simulink model "TrainModel"  (R2021a)
settings: Solver=FixedStepAuto  StartTime=0.0  StopTime=50  FixedStep=0.01  RelTol=1e-3
StopFcn:
  | if (exist('SimulinkOutput', 'file')==2)
  | SimulinkOutput(out)
  | end
settings Model: Creator=vaibhavdeshmukh  LastModifiedBy=vdmac
settings SolverCC: AlgebraicLoopSolver=TrustRegion
settings DebuggingCC: SFMachineParentedDataDiag=warning

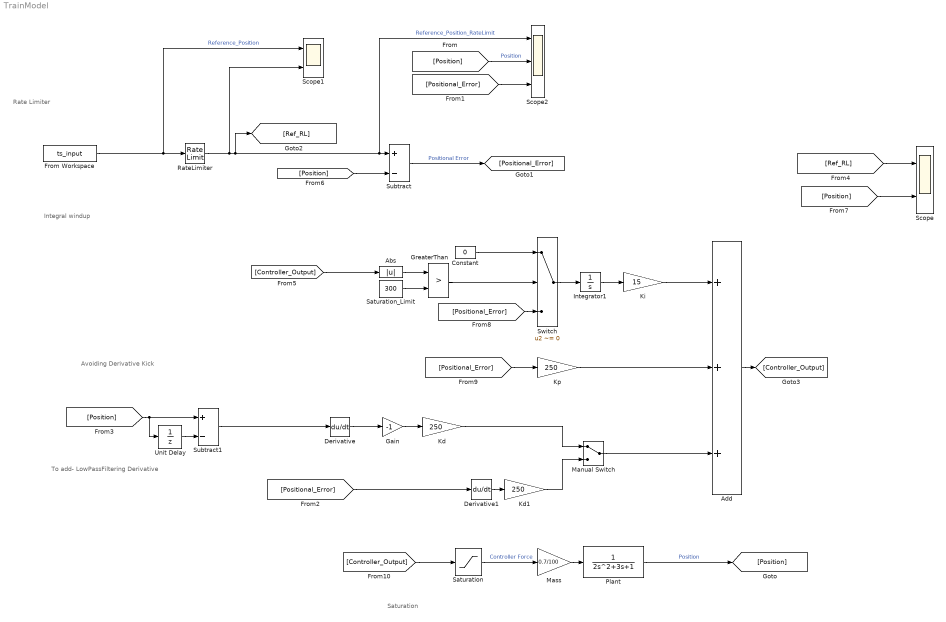
== system TrainModel ==
  note: Rate Limiter
  note: Saturation
  note: Avoiding Derivative Kick
  note: Integral windup
  note: To add- LowPassFiltering Derivative
  Abs : Abs
  Add : Sum  Inputs=+++
  Constant : Constant  Value=0
  Derivative : Derivative
  Derivative1 : Derivative
  From Workspace : FromWorkspace  VariableName=ts_input
  Gain : Gain  Gain=-1
  GreaterThan : RelationalOperator  Operator=>  OutDataTypeStr=boolean  RndMeth=Simplest
  Integrator1 : Integrator
  Kd : Gain  Gain=250
  Kd1 : Gain  Gain=250
  Ki : Gain  Gain=15
  Kp : Gain  Gain=250
  Manual Switch : ManualSwitch
  Mass : Gain  Gain=0.7/100
  Plant : TransferFcn  Denominator="[2 3  1]"
  RateLimiter : RateLimiter  RisingSlewLimit=20  FallingSlewLimit=-20  SampleTimeMode=inherited
  Saturation : Saturate  UpperLimit=10000  LowerLimit=-10000
  Saturation_Limit : Constant  Value=300
  Scope : Scope  NumInputPorts=2
  Scope1 : Scope  NumInputPorts=2
  Scope2 : Scope  NumInputPorts=3
  Subtract : Sum  Inputs=+-
  Subtract1 : Sum  Inputs=+-
  Switch : Switch  Criteria=u2 ~= 0
  Unit Delay : UnitDelay  SampleTime=-1  HasFrameUpgradeWarning=on
  wires:
  From Workspace/1 -> RateLimiter/1, Scope1/1  "Reference_Position"
  Kp/1 -> Add/2
  Mass/1 -> Plant/1
  Manual Switch/1 -> Add/3
  Switch/1 -> Integrator1/1
  Subtract/1 -> [Positional_Error]  "Positional Error"
  Plant/1 -> [Position]  "Position"
  Add/1 -> [Controller_Output]
  Saturation/1 -> Mass/1  "Controller Force"
  RateLimiter/1 -> Scope2/1, Subtract/1, [Ref_RL], Scope1/2  "Reference_Position_RateLimit"
  Derivative/1 -> Gain/1
  Unit Delay/1 -> Subtract1/2
  Saturation_Limit/1 -> GreaterThan/2
  GreaterThan/1 -> Switch/2
  Constant/1 -> Switch/1
  [Position] -> Scope2/2  "Position"
  [Positional_Error] -> Scope2/3
  Kd1/1 -> Manual Switch/2
  Kd/1 -> Manual Switch/1
  [Position] -> Subtract1/1, Unit Delay/1
  Derivative1/1 -> Kd1/1
  Ki/1 -> Add/1
  Abs/1 -> GreaterThan/1
  Integrator1/1 -> Ki/1
  [Controller_Output] -> Abs/1
  [Position] -> Subtract/2
  [Positional_Error] -> Switch/3
  [Positional_Error] -> Kp/1
  [Controller_Output] -> Saturation/1
  Gain/1 -> Kd/1
  [Position] -> Scope/2
  [Ref_RL] -> Scope/1
  [Positional_Error] -> Derivative1/1
  Subtract1/1 -> Derivative/1
